simulink model "gum_stix_fn"  (Simulink 7.1)
settings: Solver=FixedStepDiscrete  StartTime=0.0  StopTime=10.0  RelTol=1e-3
undefined symbols (not defined in the file or in its folder): DiscIntNeverNeededParam
libraries: simulink x2
settings Model: Creator=jporter  LastModifiedBy=jporter

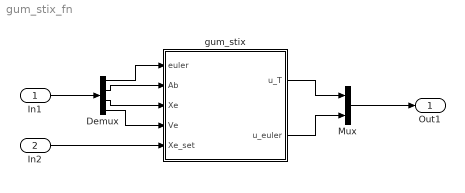
== system gum_stix_fn ==
  In1 : Inport  OutDataType=sfix(16)  OutScaling=2^0
  In2 : Inport  Port=2  OutDataType=sfix(16)  OutScaling=2^0
  Demux : Demux
  Mux : Mux  Inputs=2
  gum_stix : Subsystem
  Out1 : Outport  OutDataType=sfix(16)  OutScaling=2^0
  wires:
  Demux/1 -> gum_stix/1(euler)
  Demux/2 -> gum_stix/2(Ab)
  Demux/3 -> gum_stix/3(Xe)
  Demux/4 -> gum_stix/4(Ve)
  gum_stix/1(u_T) -> Mux/1
  gum_stix/2(u_euler) -> Mux/2
  Mux/1 -> Out1/1
  In1/1 -> Demux/1
  In2/1 -> gum_stix/5(Xe_set)

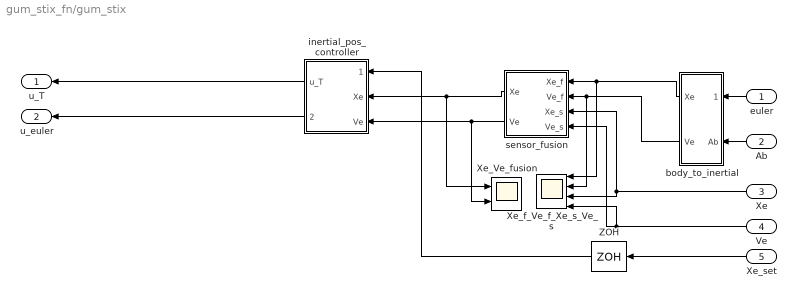
== system gum_stix_fn/gum_stix ==
  euler : Inport  Orientation=left
  Ab : Inport  Orientation=left  Port=2
  Xe : Inport  Orientation=left  Port=3
  Ve : Inport  Orientation=left  Port=4
  Xe_set : Inport  Orientation=left  Port=5
  Xe_Ve_fusion : Scope  NumInputPorts=2
      settings: YMin=-10~-5  YMax=10~5  SaveName=ScopeData2
  Xe_f_Ve_f_Xe_s_Ve_s : Scope  NumInputPorts=4
      settings: YMin=-5~-5~-5~-5  YMax=5~5~5~5  SaveName=ScopeData3
  ZOH : ZeroOrderHold  Orientation=left
  body_to_inertial : Subsystem  Orientation=left
  inertial_pos_controller : Subsystem  Orientation=left  mask{Ts=1, M=1.8263, K=7.5, K_Ve=2.5}
      mask prompts: Ts "Enter Sample Time [Ts] (seconds):"; M "Enter Mass of UAV [M] (kg):"; K "Enter Loop Gain [K]:"; K_Ve "Enter Velocity Damping Gain [K_Ve]:"
  sensor_fusion : Subsystem  Orientation=left
  u_T : Outport  Orientation=left
  u_euler : Outport  Orientation=left  Port=2
  wires:
  Xe_set/1 -> ZOH/1
  inertial_pos_controller/1(u_T) -> u_T/1
  inertial_pos_controller/2(u_euler) -> u_euler/1
  euler/1 -> body_to_inertial/1(euler)
  Ab/1 -> body_to_inertial/2(Ab)
  sensor_fusion/1(Xe) -> inertial_pos_controller/2(Xe), Xe_Ve_fusion/1
  sensor_fusion/2(Ve) -> inertial_pos_controller/3(Ve), Xe_Ve_fusion/2
  body_to_inertial/1(Xe) -> sensor_fusion/1(Xe_f), Xe_f_Ve_f_Xe_s_Ve_s/1
  body_to_inertial/2(Ve) -> sensor_fusion/2(Ve_f), Xe_f_Ve_f_Xe_s_Ve_s/2
  Xe/1 -> sensor_fusion/3(Xe_s), Xe_f_Ve_f_Xe_s_Ve_s/3
  Ve/1 -> sensor_fusion/4(Ve_s), Xe_f_Ve_f_Xe_s_Ve_s/4
  ZOH/1 -> inertial_pos_controller/1(Xe_set)

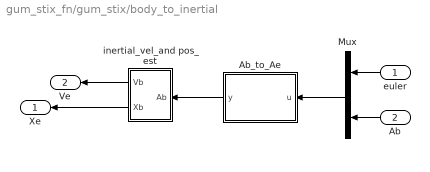
== system gum_stix_fn/gum_stix/body_to_inertial ==
  euler : Inport  Orientation=left
  Ab : Inport  Orientation=left  Port=2
  Ab_to_Ae : Stateflow chart  Orientation=left
  Mux : Mux  Orientation=left  Inputs=[3 3]
  inertial_vel_and pos_est : Subsystem  Orientation=left  mask{Ts=1}
      mask prompts: Ts "Sample Time [Ts] (seconds):"
  Xe : Outport  Orientation=left
  Ve : Outport  Orientation=left  Port=2
  wires:
  euler/1 -> Mux/1
  Ab/1 -> Mux/2
  inertial_vel_and pos_est/2(Xb) -> Xe/1
  Ab_to_Ae/1(y) -> inertial_vel_and pos_est/1(Ab)
  inertial_vel_and pos_est/1(Vb) -> Ve/1
  Mux/1 -> Ab_to_Ae/1(u)

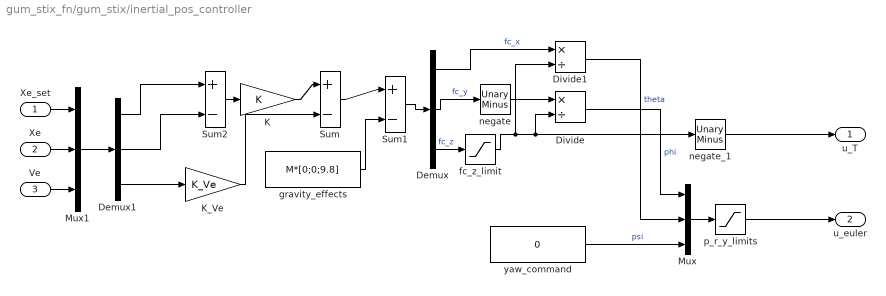
== system gum_stix_fn/gum_stix/inertial_pos_controller ==
  Xe_set : Inport
  Xe : Inport  Port=2
  Ve : Inport  Port=3
  Demux : Demux  Outputs=[1 1 1]
  Demux1 : Demux  Outputs=[3 3 3]
  Divide : Product  Inputs=*/  OutDataType=sfix(16)  OutScaling=2^-10
  Divide1 : Product  Inputs=*/  OutDataType=sfix(16)  OutScaling=2^-10
  K : Gain  Gain=K  ParameterDataType=sfix(16)  ParameterScaling=2^0  OutDataType=sfix(16)  OutScaling=2^0
  K_Ve : Gain  Gain=K_Ve  ParameterDataType=sfix(16)  ParameterScaling=2^0  OutDataType=sfix(16)  OutScaling=2^0
  Mux : Mux  Inputs=[1 1 1]
  Mux1 : Mux  Inputs=[3 3 3]
  Sum : Sum  Inputs=|+-  OutDataType=sfix(16)  OutScaling=2^0
  Sum1 : Sum  Inputs=|+-  OutDataType=sfix(16)  OutScaling=2^0
  Sum2 : Sum  Inputs=|+-  OutDataType=sfix(16)  OutScaling=2^0
  fc_z_limit : Saturate  UpperLimit=-(1/4)*9.81  LowerLimit=-4*9.81  OutDataType=sfix(16)  OutScaling=2^0
  gravity_effects : Constant  Value=M*[0;0;9.8]  OutDataType=sfix(16)  OutScaling=2^0
  negate : simulink/Math Operations/Unary Minus  DoSatur=off
  negate_1 : simulink/Math Operations/Unary Minus  DoSatur=off
  p_r_y_limits : Saturate  UpperLimit=(pi/4)*ones(3,1)  LowerLimit=-(pi/4)*ones(3,1)  OutDataType=sfix(16)  OutScaling=2^0
  yaw_command : Constant  Value=0  OutDataType=sfix(16)  OutScaling=2^0
  u_T : Outport
  u_euler : Outport  Port=2
  wires:
  fc_z_limit/1 -> Divide1/2, negate_1/1, Divide/2
  Demux1/3 -> K_Ve/1
  Mux1/1 -> Demux1/1
  Ve/1 -> Mux1/3
  Xe/1 -> Mux1/2
  Xe_set/1 -> Mux1/1
  K_Ve/1 -> Sum/2
  negate_1/1 -> u_T/1
  p_r_y_limits/1 -> u_euler/1
  Divide1/1 -> Mux/2  "theta"
  Demux/1 -> Divide1/1  "fc_x"
  Divide/1 -> Mux/1  "phi"
  negate/1 -> Divide/1
  Demux/2 -> negate/1  "fc_y"
  yaw_command/1 -> Mux/3  "psi"
  Demux/3 -> fc_z_limit/1  "fc_z"
  Mux/1 -> p_r_y_limits/1
  Sum1/1 -> Demux/1
  gravity_effects/1 -> Sum1/2
  Sum/1 -> Sum1/1
  Demux1/1 -> Sum2/1
  Demux1/2 -> Sum2/2
  Sum2/1 -> K/1
  K/1 -> Sum/1

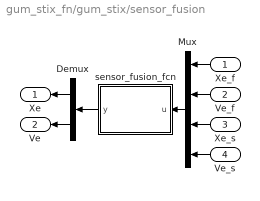
== system gum_stix_fn/gum_stix/sensor_fusion ==
  Xe_f : Inport  Orientation=left
  Ve_f : Inport  Orientation=left  Port=2
  Xe_s : Inport  Orientation=left  Port=3
  Ve_s : Inport  Orientation=left  Port=4
  Demux : Demux  Orientation=left  Outputs=[3,3]
  Mux : Mux  Orientation=left  Inputs=[3 3 3 3]
  sensor_fusion_fcn : Stateflow chart  Orientation=left
  Xe : Outport  Orientation=left
  Ve : Outport  Orientation=left  Port=2
  wires:
  Mux/1 -> sensor_fusion_fcn/1(u)
  Xe_f/1 -> Mux/1
  Demux/1 -> Xe/1
  Ve_f/1 -> Mux/2
  Demux/2 -> Ve/1
  Xe_s/1 -> Mux/3
  Ve_s/1 -> Mux/4
  sensor_fusion_fcn/1(y) -> Demux/1

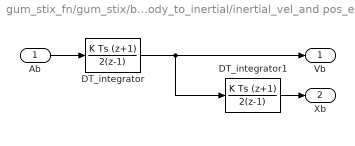
== system gum_stix_fn/gum_stix/body_to_inertial/inertial_vel_and pos_est ==
  Ab : Inport
  DT_integrator : DiscreteIntegrator  IntegratorMethod=Integration: Trapezoidal  SampleTime=Ts  OutDataType=sfix(16)  OutScaling=2^0  ICPrevOutput=DiscIntNeverNeededParam  ICPrevScaledInput=DiscIntNeverNeededParam
  DT_integrator1 : DiscreteIntegrator  IntegratorMethod=Integration: Trapezoidal  SampleTime=Ts  OutDataType=sfix(16)  OutScaling=2^0  ICPrevOutput=DiscIntNeverNeededParam  ICPrevScaledInput=DiscIntNeverNeededParam
  Vb : Outport
  Xb : Outport  Port=2
  wires:
  DT_integrator/1 -> DT_integrator1/1, Vb/1
  Ab/1 -> DT_integrator/1
  DT_integrator1/1 -> Xb/1

== matlab function gum_stix/body_to_inertial/Ab_to_Ae ==
  data: u input double size=6; y output double
function y = fcn(u)
% This block supports the Embedded MATLAB subset.
% See the help menu for details. 
phi=u(1);
theta=u(2);
psi=u(3);
c_phi=cos(phi);
c_theta=cos(theta);
c_psi=cos(psi);
s_phi=sin(phi);
s_theta=sin(theta);
s_psi=sin(psi);
R=[c_theta*c_psi, c_theta*s_psi, -s_theta;
   s_phi*s_theta*c_psi-c_phi*s_psi, s_phi*s_theta*s_psi+c_phi*c_psi, c_theta*s_phi;
   c_phi*s_theta*c_psi+s_phi*s_psi, c_phi*s_theta*s_psi-s_phi*c_psi, c_theta*c_phi];
Ae= R' * [u(4);u(5);u(6)];
[m,n]=size(u);
if m > n
    y = Ae;
else
    y = Ae';
end

== matlab function gum_stix/sensor_fusion/sensor_fusion_fcn ==
  data: u input double; y output double
function y = fcn(u)
% This block supports the Embedded MATLAB subset.
% See the help menu for details. 
persistent Xe_sh;
persistent dX;
persistent Ve_sh;
persistent dV;
Xe_f = u(1:3);
Ve_f = u(4:6);
Xe_s = u(7:9);
Ve_s = u(10:12);
if isempty(Xe_sh)
    Xe_sh = Xe_s;
    dX = Xe_f - Xe_s;
    Ve_sh = Ve_s;
    dV = Ve_f - Ve_s;
end
if Xe_s(1) ~= Xe_sh(1) || Xe_s(2) ~= Xe_sh(2) || Xe_s(3) ~= Xe_sh(3)
    Xe_sh = Xe_s;
    dX = Xe_f - Xe_s;
end
if Ve_s(1) ~= Ve_sh(1) || Ve_s(2) ~= Ve_sh(2) || Ve_s(3) ~= Ve_sh(3)
    Ve_sh = Ve_s;
    dV = Ve_f - Ve_s;
end
Xe = Xe_f - dX;
Ve = Ve_f - dV;
[m,n] = size(Xe);
if m > n
    y = [Xe;Ve];
else
    y = [Xe,Ve]';
end
